simulink model "pseudo_derivative"  (R2022a)
settings: Solver=FixedStepAuto  StartTime=0.0  StopTime=1  FixedStep=0.001  RelTol=1e-3
settings Model: Creator=김응태  LastModifiedBy=김응태

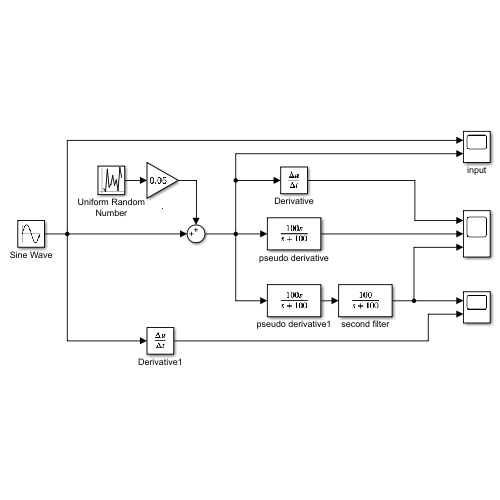
[thumbnail: Simulink's stored preview of the top-level diagram]
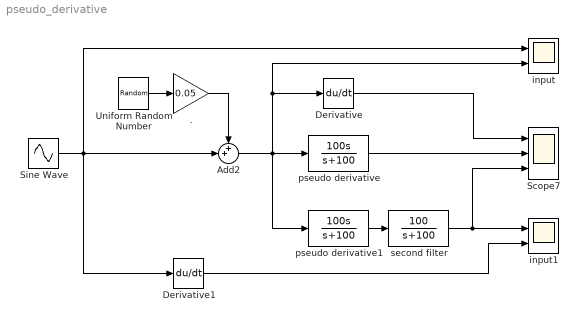
== system pseudo_derivative ==
  . : Gain  Gain=0.05
  Add2 : Sum  Inputs=++|
  Derivative : Derivative  CoefficientInTFapproximation=Inf
  Derivative1 : Derivative  CoefficientInTFapproximation=Inf
  Scope7 : Scope  NumInputPorts=3
  Sine Wave : Sin  Frequency=10  SampleTime=0
  Uniform Random Number : UniformRandomNumber
  input : Scope  NumInputPorts=2
  input1 : Scope  NumInputPorts=2
  pseudo derivative : TransferFcn  Numerator=[100 0]  Denominator="[1  100]"
  pseudo derivative1 : TransferFcn  Numerator=[100 0]  Denominator="[1  100]"
  second filter : TransferFcn  Numerator=100  Denominator="[1  100]"
  wires:
  Sine Wave/1 -> input/1, Derivative1/1, Add2/2
  Uniform Random Number/1 -> ./1
  ./1 -> Add2/1
  pseudo derivative1/1 -> second filter/1
  second filter/1 -> input1/1, Scope7/3
  Add2/1 -> input/2, Derivative/1, pseudo derivative1/1, pseudo derivative/1
  Derivative/1 -> Scope7/1
  pseudo derivative/1 -> Scope7/2
  Derivative1/1 -> input1/2
